simulink model "thermostat_simulink"  (R2019b)
settings: Solver=VariableStepAuto  StartTime=0.0  StopTime=800  RelTol=1e-3
settings Model: Creator=Δημήτρης  LastModifiedBy=Εμμανουήλ

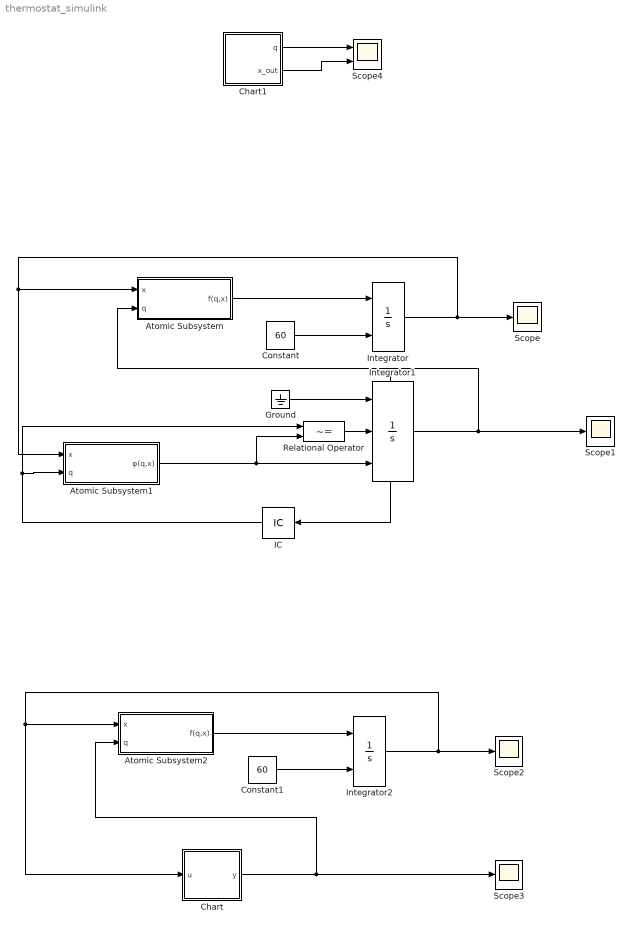
== system thermostat_simulink ==
  Atomic Subsystem : Subsystem  TreatAsAtomicUnit=on
  Atomic Subsystem1 : Subsystem  TreatAsAtomicUnit=on
  Atomic Subsystem2 : Subsystem  TreatAsAtomicUnit=on
  Chart : Stateflow chart  BlockKeywords=__PRM__SERIALIZED__DATA__:Stateflow Chart,Stateflow Diagram  TreatAsAtomicUnit=on
  Chart1 : Stateflow chart  BlockKeywords=__PRM__SERIALIZED__DATA__:Stateflow Chart,Stateflow Diagram  TreatAsAtomicUnit=on
  Constant : Constant  Value=60
  Constant1 : Constant  Value=60
  Ground : Ground
  IC : InitialCondition
  Integrator : Integrator  InitialConditionSource=external
  Integrator1 : Integrator  ExternalReset=rising  InitialConditionSource=external  ShowStatePort=on
  Integrator2 : Integrator  InitialConditionSource=external
  Relational Operator : RelationalOperator  Operator=~=  OutDataTypeStr=boolean  RndMeth=Simplest
  Scope{,1..3} (4 alike) : Scope
  Scope4 : Scope  NumInputPorts=2
  wires:
  Constant/1 -> Integrator/2
  Atomic Subsystem/1("f(q,x) ") -> Integrator/1
  Integrator1/State -> IC/1
  Atomic Subsystem1/1(φ(q,x)) -> Relational Operator/2, Integrator1/3
  Relational Operator/1 -> Integrator1/2
  Ground/1 -> Integrator1/1
  IC/1 -> Relational Operator/1, Atomic Subsystem1/2(q)
  Integrator1/1 -> Scope1/1, Atomic Subsystem/2(q)
  Integrator/1 -> Atomic Subsystem/1(x), Atomic Subsystem1/1(x), Scope/1
  Integrator2/1 -> Scope2/1, Chart/1(u), Atomic Subsystem2/1(x)
  Atomic Subsystem2/1("f(q,x) ") -> Integrator2/1
  Constant1/1 -> Integrator2/2
  Chart/1(y) -> Atomic Subsystem2/2(q), Scope3/1
  Chart1/2(x_out) -> Scope4/2
  Chart1/1(q) -> Scope4/1

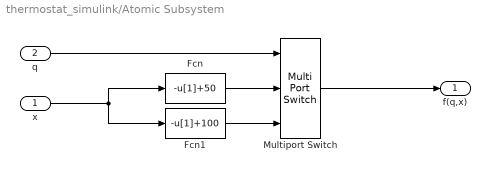
== system thermostat_simulink/Atomic Subsystem ==
  x : Inport
  q : Inport  Port=2
  Fcn : Fcn  Expr=-u[1]+50
  Fcn1 : Fcn  Expr=-u[1]+100
  Multiport Switch : MultiPortSwitch  DataPortOrder=Zero-based contiguous  Inputs=2  zeroidx=on
  "f(q,x) " : Outport
  wires:
  Fcn/1 -> Multiport Switch/2
  Fcn1/1 -> Multiport Switch/3
  q/1 -> Multiport Switch/1
  x/1 -> Fcn/1, Fcn1/1
  Multiport Switch/1 -> "f(q,x) "/1

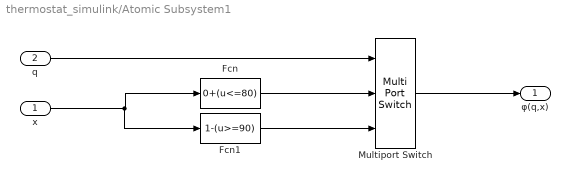
== system thermostat_simulink/Atomic Subsystem1 ==
  x : Inport
  q : Inport  Port=2
  Fcn : Fcn  Expr=0+(u<=80)
  Fcn1 : Fcn  Expr=1-(u>=90)
  Multiport Switch : MultiPortSwitch  DataPortOrder=Zero-based contiguous  Inputs=2  zeroidx=on
  φ(q,x) : Outport
  wires:
  Multiport Switch/1 -> φ(q,x)/1
  Fcn1/1 -> Multiport Switch/3
  Fcn/1 -> Multiport Switch/2
  x/1 -> Fcn1/1, Fcn/1
  q/1 -> Multiport Switch/1

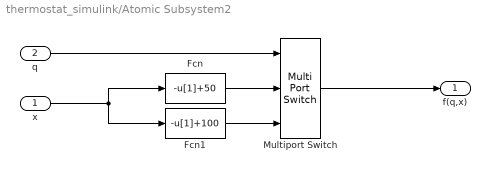
== system thermostat_simulink/Atomic Subsystem2 ==
  x : Inport
  q : Inport  Port=2
  Fcn : Fcn  Expr=-u[1]+50
  Fcn1 : Fcn  Expr=-u[1]+100
  Multiport Switch : MultiPortSwitch  DataPortOrder=Zero-based contiguous  Inputs=2  zeroidx=on
  "f(q,x) " : Outport
  wires:
  Multiport Switch/1 -> "f(q,x) "/1
  x/1 -> Fcn1/1, Fcn/1
  q/1 -> Multiport Switch/1
  Fcn1/1 -> Multiport Switch/3
  Fcn/1 -> Multiport Switch/2

== stateflow chart thermostat_simulink/Chart1 ==
  settings: updateMethod=CONTINUOUS  executeAtInitialization=1  initializeOutput=1
  state ON
    du:
    x_dot=-x+100;
    %outputs
    x_out=x;
    q=1;
  state OFF
    du:
    x_dot=-x+50;
    %outputs
    x_out=x;
    q=2;
  ON -> OFF : [x>=90]
  (default) -> ON : {x=20;}
  OFF -> ON : [x<=80]
  data: q output; x_out output; x local
  data x settings: updateMethod=SF_CONTINUOUS_TIME_DATA

== stateflow chart thermostat_simulink/Chart ==
  state on
    entry:y=1;
  state off
    entry:y=0;
  (default) -> on
  on -> off : [u>=90]
  off -> on : [u<=80]
  data: u input; y output
